simulink model "pid_fuzzy_controller"  (Simulink 6.3)
settings: Solver=ode45  StartTime=0.0  StopTime=40.0  MaxStep=0.1  MinStep=0.001  RelTol=0.001  AbsTol=0.01
libraries: fuzblock x1
settings Model: LastModifiedBy=Administrator
settings SolverCC: InitialStep=0.001
settings OptimizationCC: BooleanDataType=off
settings DebuggingCC: SolverPrmCheckMsg=none
settings HardwareCC: TargetUnknown=on

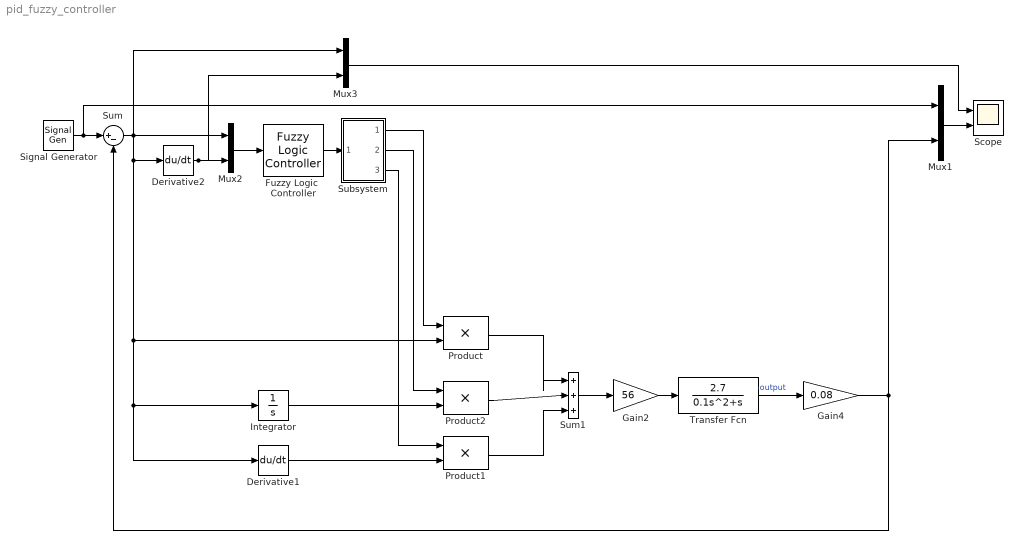
== system pid_fuzzy_controller ==
  Derivative1 : Derivative
  Derivative2 : Derivative
  Fuzzy Logic  Controller : fuzblock/Fuzzy Logic  Controller  fis=fuzzy_pid
  Gain2 : Gain  Gain=56  SaturateOnIntegerOverflow=on
  Gain4 : Gain  Gain=0.08  SaturateOnIntegerOverflow=on
  Integrator : Integrator
  Mux1 : Mux  Inputs=2
  Mux2 : Mux  Inputs=2
  Mux3 : Mux  Inputs=2
  Product : Product  SaturateOnIntegerOverflow=on  RndMeth=Zero  InputSameDT=on
  Product1 : Product  SaturateOnIntegerOverflow=on  RndMeth=Zero  InputSameDT=on
  Product2 : Product  SaturateOnIntegerOverflow=on  RndMeth=Zero  InputSameDT=on
  Scope : Scope  NumInputPorts=2
      settings: TimeRange=10  YMin=0~0.25  YMax=5.5~0.39  MaxDataPoints=10000
  Signal Generator : SignalGenerator  Amplitude=10  Frequency=5  Units=rad/sec
  Subsystem : Subsystem
  Sum : Sum  Inputs=|+-  SaturateOnIntegerOverflow=on  InputSameDT=on
  Sum1 : Sum  Inputs=|+++  SaturateOnIntegerOverflow=on  InputSameDT=on
  Transfer Fcn : TransferFcn  Numerator=[2.7]  Denominator=[0.1 1 0]
  wires:
  Transfer Fcn/1 -> Gain4/1  "output"
  Gain2/1 -> Transfer Fcn/1
  Signal Generator/1 -> Sum/1, Mux1/1
  Mux1/1 -> Scope/2
  Derivative1/1 -> Product1/2
  Integrator/1 -> Product2/2
  Product/1 -> Sum1/1
  Sum1/1 -> Gain2/1
  Sum/1 -> Mux2/1, Derivative2/1, Derivative1/1, Integrator/1, Product/2, Mux3/1
  Derivative2/1 -> Mux2/2, Mux3/2
  Mux2/1 -> Fuzzy Logic  Controller/1
  Fuzzy Logic  Controller/1 -> Subsystem/1(In1)
  Product2/1 -> Sum1/2
  Product1/1 -> Sum1/3
  Gain4/1 -> Mux1/2, Sum/2
  Mux3/1 -> Scope/1
  Subsystem/1(Out1) -> Product/1
  Subsystem/2(Out2) -> Product2/1
  Subsystem/3(Out3) -> Product1/1

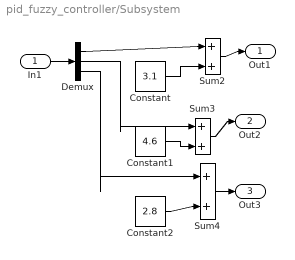
== system pid_fuzzy_controller/Subsystem ==
  In1 : Inport
  Constant : Constant  Value=3.1
  Constant1 : Constant  Value=4.6
  Constant2 : Constant  Value=2.8
  Demux : Demux  Outputs=3
  Sum2 : Sum  Inputs=|++  SaturateOnIntegerOverflow=on  InputSameDT=on
  Sum3 : Sum  Inputs=|++  SaturateOnIntegerOverflow=on  InputSameDT=on
  Sum4 : Sum  Inputs=|++  SaturateOnIntegerOverflow=on  InputSameDT=on
  Out1 : Outport
  Out2 : Outport  Port=2
  Out3 : Outport  Port=3
  wires:
  Demux/1 -> Sum2/1
  Demux/2 -> Sum3/1
  Demux/3 -> Sum4/1
  Constant/1 -> Sum2/2
  Constant1/1 -> Sum3/2
  Constant2/1 -> Sum4/2
  Sum2/1 -> Out1/1
  In1/1 -> Demux/1
  Sum3/1 -> Out2/1
  Sum4/1 -> Out3/1
